simulink library "Disabled_lib"  (R2023b)
settings: Solver=VariableStepAuto  StartTime=0.0  StopTime=10.0  RelTol=1e-3
undefined symbols (not defined in the file): Spline_Num_Poses_default, Spline_Ref_Poses_default
settings Model: Creator=FIRSTMentor  LastModifiedBy=ander

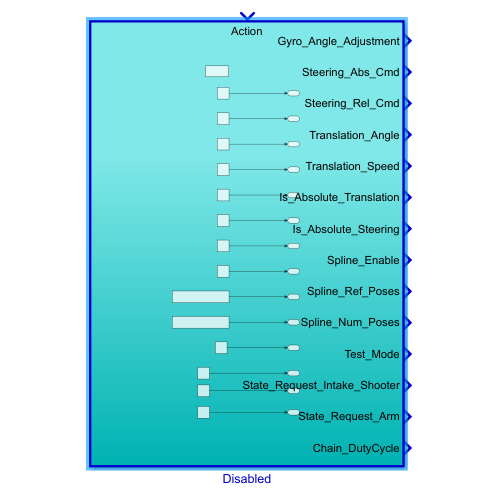
[thumbnail: Simulink's stored preview of the top-level diagram]
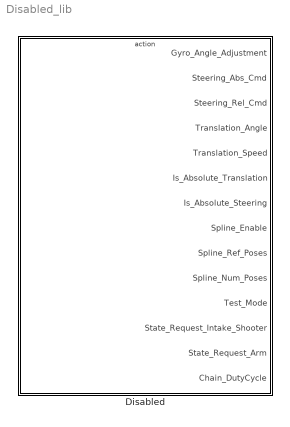
== system Disabled_lib ==
  Disabled : Subsystem  TreatAsAtomicUnit=on

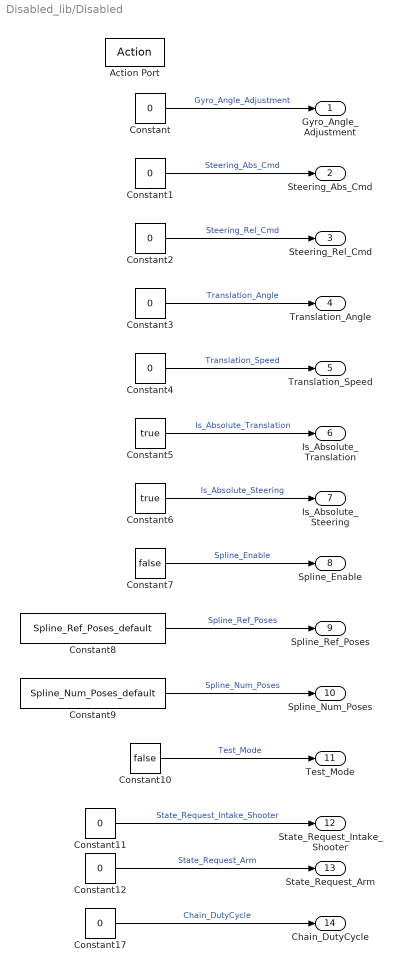
== system Disabled_lib/Disabled ==
  Action Port : ActionPort
  Constant{,1..4,11..12,17} (8 alike) : Constant  Value=0
  Constant10 : Constant  Value=false  OutDataTypeStr=boolean
  Constant5 : Constant  Value=true
  Constant6 : Constant  Value=true
  Constant7 : Constant  Value=false  OutDataTypeStr=boolean
  Constant8 : Constant  Value=Spline_Ref_Poses_default
  Constant9 : Constant  Value=Spline_Num_Poses_default  OutDataTypeStr=double
  Gyro_Angle_Adjustment : Outport
  Steering_Abs_Cmd : Outport  Port=2
  Steering_Rel_Cmd : Outport  Port=3
  Translation_Angle : Outport  Port=4
  Translation_Speed : Outport  Port=5
  Is_Absolute_Translation : Outport  Port=6
  Is_Absolute_Steering : Outport  Port=7
  Spline_Enable : Outport  Port=8
  Spline_Ref_Poses : Outport  Port=9
  Spline_Num_Poses : Outport  Port=10
  Test_Mode : Outport  Port=11
  State_Request_Intake_Shooter : Outport  Port=12
  State_Request_Arm : Outport  Port=13
  Chain_DutyCycle : Outport  Port=14
  wires:
  Constant/1 -> Gyro_Angle_Adjustment/1  "Gyro_Angle_Adjustment"
  Constant1/1 -> Steering_Abs_Cmd/1  "Steering_Abs_Cmd"
  Constant2/1 -> Steering_Rel_Cmd/1  "Steering_Rel_Cmd"
  Constant3/1 -> Translation_Angle/1  "Translation_Angle"
  Constant4/1 -> Translation_Speed/1  "Translation_Speed"
  Constant5/1 -> Is_Absolute_Translation/1  "Is_Absolute_Translation"
  Constant6/1 -> Is_Absolute_Steering/1  "Is_Absolute_Steering"
  Constant7/1 -> Spline_Enable/1  "Spline_Enable"
  Constant8/1 -> Spline_Ref_Poses/1  "Spline_Ref_Poses"
  Constant9/1 -> Spline_Num_Poses/1  "Spline_Num_Poses"
  Constant10/1 -> Test_Mode/1  "Test_Mode"
  Constant12/1 -> State_Request_Arm/1  "State_Request_Arm"
  Constant11/1 -> State_Request_Intake_Shooter/1  "State_Request_Intake_Shooter"
  Constant17/1 -> Chain_DutyCycle/1  "Chain_DutyCycle"
